simulink model "electrical_model"  (R2016a)
settings: Solver=VariableStepAuto  StartTime=0.0  StopTime=5  FixedStep=Ts  RelTol=1e-3
values from neighbouring files (symbols this model uses):
  Ts = 1    [MPC.m]
undefined symbols (not defined in the file or in its folder): Continuous, DiscIntNeverNeededParam, F, Li, ri, spsPMSynchronousMachineModel, w_g
libraries: powerlib x11, dspsrcs4 x6, powerlib_meascontrol x2, mpclib x1
settings Model: Creator=syf  LastModifiedBy=syf
settings SolverCC: AutoInsertRateTranBlk=on

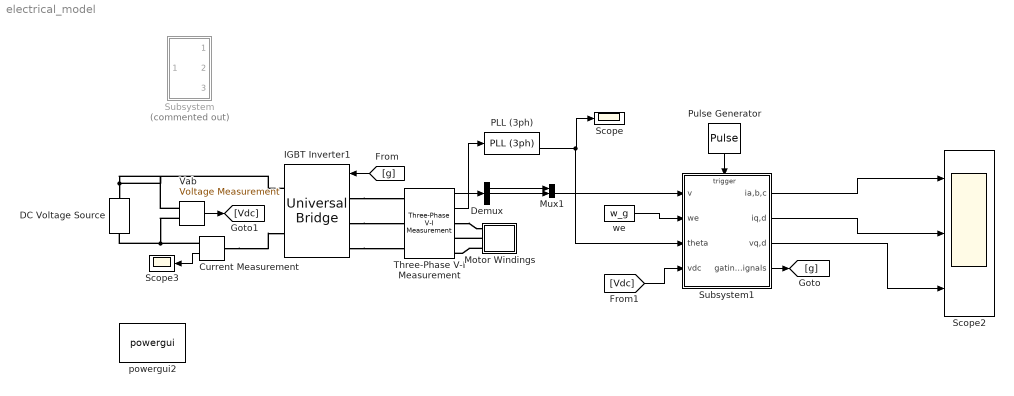
== system electrical_model ==
  Current Measurement : powerlib/Measurements/Current Measurement  PhasorSimulation=off  OutputType=Complex  PSBequivalent=0
  DC Voltage Source : powerlib/Electrical Sources/DC Voltage Source  Amplitude=540  Measurements=None
  Demux : Demux  Outputs=3
  IGBT Inverter1 : powerlib/Power Electronics/Universal Bridge  Arms=3  SnubberResistance=1e6  SnubberCapacitance=1e-9  Device=IGBT / Diodes  Ron=1e-3  Lon=0  ForwardVoltages="[  0.8  0.8  ]"  ForwardVoltage=.8  GTOparameters=[ 1e-6 , 1e-6 ]  IGBTparameters=[ 1e-6 , 2e-6 ]  Measurements=All voltages and currents  Measurements_2=None  converterType=Rectifier
  Motor Windings : Subsystem
  Mux1 : Mux  Inputs=2
  PLL (3ph) : powerlib_meascontrol/PLL/PLL (3ph)  Fmin=45  Par_Init=[0, 60]  ParK=[180, 3200, 1]  TcD=1e-4  MaxRateChangeFreq=12  FilterCutOffFreq=25  Ts=0  AGC=on
  Pulse Generator : DiscretePulseGenerator  PulseType=Time based  Period=Ts  PulseWidth=20
  Scope : Scope
  Scope2 : Scope  NumInputPorts=3
  Scope3 : Scope
  Subsystem : Subsystem  Commented=on
  Subsystem1 : Subsystem
  Three-Phase V-I Measurement : powerlib/Measurements/Three-Phase V-I Measurement  VoltageMeasurement=phase-to-phase  SetLabelV=off  LabelV=Vabc  Vpu=off  VpuLL=off  CurrentMeasurement=yes  SetLabelI=off  LabelI=Iabc  Ipu=off  Pbase=100e6  Vbase=500e3  OutputType=Complex  PhasorSimulation=off  PSBequivalent=0
  Vab : powerlib/Measurements/Voltage Measurement  Tag=PoWeRsYsTeMmEaSuReMeNt  PhasorSimulation=off  OutputType=Magnitude  PSBequivalent=0
  powergui2 : powerlib/powergui  Priority=1  SimulationMode=Continuous  SolverType=Backward Euler  SampleTime=Ts  frequency=60  SPID=off  DisableSnubberDevices=off  DisableRonSwitches=off  DisableVfSwitches=off  SwTol=0  DisplayEquations=off  Interpol=off  ExternalGateDelay=off  methode=off  Ts=10  FunctionMessages=off  echomessages=off  HookPort=off  EnableUseOfTLC=off  x0status=blocks  frequencyindice=0  Pbase=100e6  ErrMax=1e-4  Iterations=50  UnitsV=kV  UnitsW=MW  buscounter=0  RestoreLinks=warning  ResistiveCurrentMeasurement=off  Frange=[0:2:500]  Ylog=off  Xlog=on  ShowGrid=off  save=off  variable=ZData  structure=0  ZoomFFT=off  StartTime=0.0  cycles=1  DisplayStyle=1  fundamental=60  FreqAxis=off  MaxFrequency=1000  frequencyindicesteady=1  RmsSteady=1  display=off
  we : Constant  Value=w_g
  wires:
  Three-Phase V-I Measurement/1 -> Demux/1
  Demux/1 -> Mux1/1
  Demux/2 -> Mux1/2
  Vab/1 -> [Vdc]
  Current Measurement/1 -> Scope3/1
  Three-Phase V-I Measurement/2 -> PLL (3ph)/1
  PLL (3ph)/2 -> Subsystem1/3(theta), Scope/1
  [g] -> IGBT Inverter1/1
  Pulse Generator/1 -> Subsystem1/Trigger
  we/1 -> Subsystem1/2(we)
  [Vdc] -> Subsystem1/4(vdc)
  Subsystem1/4(gating signals) -> [g]
  Mux1/1 -> Subsystem1/1(v)
  Subsystem1/1(ia,b,c) -> Scope2/1
  Subsystem1/2(iq,d) -> Scope2/2
  Subsystem1/3(vq,d) -> Scope2/3
  connections:
  Current Measurement/RConn1 -- Vab/LConn2 -- DC Voltage Source/LConn1
  DC Voltage Source/RConn1 -- IGBT Inverter1/RConn1 -- Vab/LConn1
  Current Measurement/LConn1 -- IGBT Inverter1/RConn2
  IGBT Inverter1/LConn1 -- Three-Phase V-I Measurement/LConn1
  IGBT Inverter1/LConn2 -- Three-Phase V-I Measurement/LConn2
  IGBT Inverter1/LConn3 -- Three-Phase V-I Measurement/LConn3
  Three-Phase V-I Measurement/RConn1 -- Motor Windings/LConn1
  Motor Windings/LConn2 -- Three-Phase V-I Measurement/RConn2
  Motor Windings/LConn3 -- Three-Phase V-I Measurement/RConn3

== system electrical_model/Motor Windings ==
  phasea : powerlib/Elements/Series RLC Branch  LConnTagsString=__new0  RConnTagsString=__new0  BranchType=RL  Resistance=8e-3  Inductance=2.07e-3  SetiL0=off  InitialCurrent=0  Capacitance=0  Setx0=off  InitialVoltage=0  Measurements=None
  phaseb : powerlib/Elements/Series RLC Branch  LConnTagsString=__new0  RConnTagsString=__new0  BranchType=RL  Resistance=8e-3  Inductance=2.07e-3  SetiL0=off  InitialCurrent=0  Capacitance=0  Setx0=off  InitialVoltage=0  Measurements=None
  phasec : powerlib/Elements/Series RLC Branch  LConnTagsString=__new0  RConnTagsString=__new0  BranchType=RL  Resistance=8e-3  Inductance=2.07e-3  SetiL0=off  InitialCurrent=0  Capacitance=0  Setx0=off  InitialVoltage=0  Measurements=None
  A : PMIOPort  Port=1  Side=Left
  B : PMIOPort  Port=2  Side=Left
  C : PMIOPort  Port=3  Side=Left
  connections:
  phasea/RConn1 -- phasec/RConn1 -- phaseb/RConn1
  phaseb/LConn1 -- B/RConn1
  A/RConn1 -- phasea/LConn1
  phasec/LConn1 -- C/RConn1

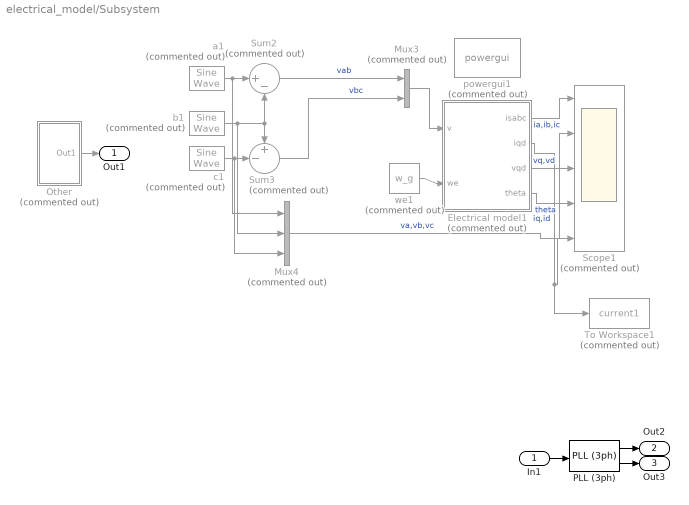
== system electrical_model/Subsystem ==
  In1 : Inport
  Electrical model1 : Subsystem  Commented=on  AncestorBlock=spsPMSynchronousMachineModel/Continuous
  Mux3 : Mux  Commented=on  Inputs=2
  Mux4 : Mux  Commented=on  Inputs=3
  Other : Subsystem  Commented=on
  PLL (3ph) : powerlib_meascontrol/PLL/PLL (3ph)  Fmin=45  Par_Init=[0, 60]  ParK=[180, 3200, 1]  TcD=1e-4  MaxRateChangeFreq=12  FilterCutOffFreq=25  Ts=0  AGC=on
  Scope1 : Scope  Commented=on  NumInputPorts=5
  Sum2 : Sum  Commented=on  Inputs=|+-
  Sum3 : Sum  Commented=on  Inputs=+-|
  To Workspace1 : ToWorkspace  Commented=on  VariableName=current1  SampleTime=-1
  a1 : dspsrcs4/Sine Wave  Commented=on  Amplitude=200  Frequency=w_g/(2*pi)  Phase=0  SampleMode=Discrete  OutComplex=Real  CompMethod=Trigonometric fcn  TableSize=Speed  SampleTime=Ts  SamplesPerFrame=1  ResetState=Restart at time zero  OutputFrames=off  dataType=double  wordLen=16  udDataType=sfix(16)  fracBitsMode=Best precision  numFracBits=15  OutDataTypeStr=double  LastOutDataTypeStr=double
  b1 : dspsrcs4/Sine Wave  Commented=on  Amplitude=200  Frequency=w_g/(2*pi)  Phase=2*pi/3  SampleMode=Discrete  OutComplex=Real  CompMethod=Trigonometric fcn  TableSize=Speed  SampleTime=Ts  SamplesPerFrame=1  ResetState=Restart at time zero  OutputFrames=off  dataType=double  wordLen=16  udDataType=sfix(16)  fracBitsMode=Best precision  numFracBits=15  OutDataTypeStr=double  LastOutDataTypeStr=double
  c1 : dspsrcs4/Sine Wave  Commented=on  Amplitude=200  Frequency=w_g/(2*pi)  Phase=-2*pi/3  SampleMode=Discrete  OutComplex=Real  CompMethod=Trigonometric fcn  TableSize=Speed  SampleTime=Ts  SamplesPerFrame=1  ResetState=Restart at time zero  OutputFrames=off  dataType=double  wordLen=16  udDataType=sfix(16)  fracBitsMode=Best precision  numFracBits=15  OutDataTypeStr=double  LastOutDataTypeStr=double
  powergui1 : powerlib/powergui  Priority=1  Commented=on  SimulationMode=Discrete  SolverType=Backward Euler  SampleTime=Ts  frequency=60  SPID=off  DisableSnubberDevices=off  DisableRonSwitches=off  DisableVfSwitches=off  SwTol=0  DisplayEquations=off  Interpol=off  ExternalGateDelay=off  methode=off  Ts=10  FunctionMessages=off  echomessages=off  HookPort=off  EnableUseOfTLC=off  x0status=blocks  frequencyindice=60  Pbase=100e6  ErrMax=1e-4  Iterations=50  UnitsV=kV  UnitsW=MW  buscounter=0  RestoreLinks=warning  ResistiveCurrentMeasurement=off  Frange=[0:2:500]  Ylog=off  Xlog=on  ShowGrid=off  save=off  variable=ZData  structure=0  ZoomFFT=off  StartTime=0.0  cycles=1  DisplayStyle=1  fundamental=60  FreqAxis=off  MaxFrequency=1000  frequencyindicesteady=1  RmsSteady=1  display=off
  we1 : Constant  Commented=on  Value=w_g
  Out1 : Outport
  Out2 : Outport  Port=2
  Out3 : Outport  Port=3
  wires:
  PLL (3ph)/2 -> Out3/1
  PLL (3ph)/1 -> Out2/1
  Other/1(Out1) -> Out1/1
  In1/1 -> PLL (3ph)/1
  we1/1 -> Electrical model1/2(we)
  Mux3/1 -> Electrical model1/1(v)
  Sum2/1 -> Mux3/1  "vab"
  Sum3/1 -> Mux3/2  "vbc"
  Electrical model1/1(isabc) -> Scope1/1  "ia,ib,ic"
  a1/1 -> Sum2/1, Mux4/1
  Electrical model1/2(iqd) -> To Workspace1/1, Scope1/5  "iq,id"
  c1/1 -> Sum3/2, Mux4/3
  Mux4/1 -> Scope1/2  "va,vb,vc"
  b1/1 -> Sum2/2, Sum3/1, Mux4/2
  Electrical model1/4(theta) -> Scope1/4  "theta"
  Electrical model1/3(vqd) -> Scope1/3  "vq,vd"

== system electrical_model/Subsystem1 ==
  v : Inport
  we : Inport  Port=2
  theta : Inport  Port=3
  vdc : Inport  Port=4
  Trigger : TriggerPort  VariantControl=Variant  PortDimensions=1
  Electrical model2 : Subsystem  AncestorBlock=spsPMSynchronousMachineModel/Continuous
  ia,b,c : Outport
  iq,d : Outport  Port=2
  vq,d : Outport  Port=3
  gating signals : Outport  Port=4
  wires:
  v/1 -> Electrical model2/1(v)
  we/1 -> Electrical model2/2(we)
  theta/1 -> Electrical model2/3(theta)
  Electrical model2/1(isabc) -> ia,b,c/1  "ia,ib,ic"
  Electrical model2/3(vqd) -> vq,d/1  "vq,vd"
  Electrical model2/4(Pulses) -> gating signals/1
  vdc/1 -> Electrical model2/4(Vdc)
  Electrical model2/2(iqd) -> iq,d/1  "iq,id"

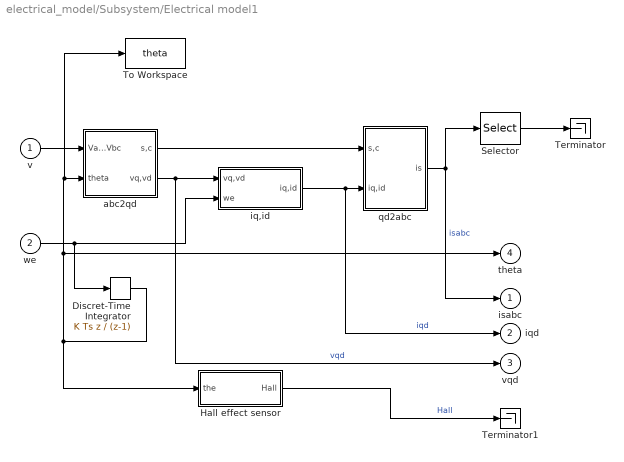
== system electrical_model/Subsystem/Electrical model1 ==
  v : Inport
  we : Inport  Port=2
  Discret-Time Integrator : DiscreteIntegrator  IntegratorMethod=Integration: Backward Euler  gainval=1  InitialConditionSetting=State (most efficient)  SampleTime=Ts  ICPrevOutput=DiscIntNeverNeededParam  ICPrevScaledInput=DiscIntNeverNeededParam
  Hall effect sensor : Subsystem
  Selector : Selector  InputPortWidth=3  IndexOptions=Index vector (dialog)  Indices=1:2  OutputSizes=1
  Terminator : Terminator
  Terminator1 : Terminator
  To Workspace : ToWorkspace  VariableName=theta  SampleTime=-1
      settings: Save2DSignal=2-D array (concatenate along first dimension)
  abc2qd : Subsystem
  iq,id : Subsystem
  qd2abc : Subsystem
  isabc : Outport  InitialOutput=0
  iqd : Outport  Port=2  InitialOutput=0
  vqd : Outport  Port=3  InitialOutput=0
  theta : Outport  Port=4  InitialOutput=0
  wires:
  we/1 -> Discret-Time Integrator/1, iq,id/2(we)
  Discret-Time Integrator/1 -> Hall effect sensor/1(the), theta/1, abc2qd/2(theta), To Workspace/1
  abc2qd/2(vq,vd) -> iq,id/1(vq,vd), vqd/1  "vqd"
  abc2qd/1(s,c) -> qd2abc/1(s,c)
  v/1 -> abc2qd/1(Vab,Vbc)
  iq,id/1(iq,id) -> qd2abc/2(iq,id), iqd/1  "iqd"
  qd2abc/1(is) -> Selector/1, isabc/1  "isabc"
  Selector/1 -> Terminator/1
  Hall effect sensor/1(Hall) -> Terminator1/1  "Hall"

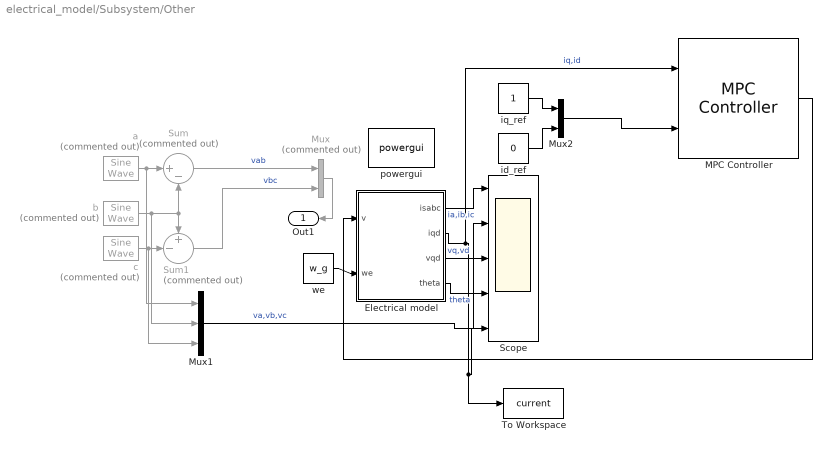
== system electrical_model/Subsystem/Other ==
  Electrical model : Subsystem  AncestorBlock=spsPMSynchronousMachineModel/Continuous
  MPC Controller : mpclib/MPC Controller  SCDEnableBlockLinearizationSpecification=on  is_multiple=0  enable_value=0  return_u0=off  ref_from_ws=off  ref_signal_name=[]  ref_preview=off  md_from_ws=off  md_signal_name=[]  md_preview=off  from_project=off  project_file=MPCtask.mat  md_inport=off  mv_inport=off  cost_outport=off  return_sequence=off  return_qpstatus=off  return_state=off  state_inport=off  lims_inport=off  ywt_inport=off  is_designfromscratch=0  uwt_inport=off  duwt_inport=off  rhoeps_inport=off  uref_inport=off  n_ts=1  n_mv=2  n_md=1  n_ud=0  n_mo=2  n_uo=0  BlockDataType=double  SampleTimeInherited=off  switch_inport=off
  Mux : Mux  Commented=on  Inputs=2
  Mux1 : Mux  Inputs=3
  Mux2 : Mux  Inputs=2
  Scope : Scope  NumInputPorts=5
  Sum : Sum  Commented=on  Inputs=|+-
  Sum1 : Sum  Commented=on  Inputs=+-|
  To Workspace : ToWorkspace  VariableName=current  SampleTime=-1
  a : dspsrcs4/Sine Wave  Commented=on  Amplitude=200  Frequency=w_g/(2*pi)  Phase=0  SampleMode=Discrete  OutComplex=Real  CompMethod=Trigonometric fcn  TableSize=Speed  SampleTime=Ts  SamplesPerFrame=1  ResetState=Restart at time zero  OutputFrames=off  dataType=double  wordLen=16  udDataType=sfix(16)  fracBitsMode=Best precision  numFracBits=15  OutDataTypeStr=double  LastOutDataTypeStr=double
  b : dspsrcs4/Sine Wave  Commented=on  Amplitude=200  Frequency=w_g/(2*pi)  Phase=2*pi/3  SampleMode=Discrete  OutComplex=Real  CompMethod=Trigonometric fcn  TableSize=Speed  SampleTime=Ts  SamplesPerFrame=1  ResetState=Restart at time zero  OutputFrames=off  dataType=double  wordLen=16  udDataType=sfix(16)  fracBitsMode=Best precision  numFracBits=15  OutDataTypeStr=double  LastOutDataTypeStr=double
  c : dspsrcs4/Sine Wave  Commented=on  Amplitude=200  Frequency=w_g/(2*pi)  Phase=-2*pi/3  SampleMode=Discrete  OutComplex=Real  CompMethod=Trigonometric fcn  TableSize=Speed  SampleTime=Ts  SamplesPerFrame=1  ResetState=Restart at time zero  OutputFrames=off  dataType=double  wordLen=16  udDataType=sfix(16)  fracBitsMode=Best precision  numFracBits=15  OutDataTypeStr=double  LastOutDataTypeStr=double
  id_ref : Constant  Value=0
  iq_ref : Constant
  powergui : powerlib/powergui  Priority=1  SimulationMode=Discrete  SolverType=Backward Euler  SampleTime=Ts  frequency=60  SPID=off  DisableSnubberDevices=off  DisableRonSwitches=off  DisableVfSwitches=off  SwTol=0  DisplayEquations=off  Interpol=off  ExternalGateDelay=off  methode=off  Ts=10  FunctionMessages=off  echomessages=off  HookPort=off  EnableUseOfTLC=off  x0status=blocks  frequencyindice=60  Pbase=100e6  ErrMax=1e-4  Iterations=50  UnitsV=kV  UnitsW=MW  buscounter=0  RestoreLinks=warning  ResistiveCurrentMeasurement=off  Frange=[0:2:500]  Ylog=off  Xlog=on  ShowGrid=off  save=off  variable=ZData  structure=0  ZoomFFT=off  StartTime=0.0  cycles=1  DisplayStyle=1  fundamental=60  FreqAxis=off  MaxFrequency=1000  frequencyindicesteady=1  RmsSteady=1  display=off
  we : Constant  Value=w_g
  Out1 : Outport
  wires:
  Electrical model/4(theta) -> Scope/4  "theta"
  Mux2/1 -> MPC Controller/2
  iq_ref/1 -> Mux2/1
  we/1 -> Electrical model/2(we)
  Sum/1 -> Mux/1  "vab"
  Electrical model/1(isabc) -> Scope/1  "ia,ib,ic"
  Electrical model/3(vqd) -> Scope/3  "vq,vd"
  Mux/1 -> Out1/1
  a/1 -> Mux1/1, Sum/1
  Electrical model/2(iqd) -> MPC Controller/1, Scope/5, To Workspace/1  "iq,id"
  b/1 -> Mux1/2, Sum1/1, Sum/2
  Sum1/1 -> Mux/2  "vbc"
  c/1 -> Mux1/3, Sum1/2
  Mux1/1 -> Scope/2  "va,vb,vc"
  MPC Controller/1 -> Electrical model/1(v)
  id_ref/1 -> Mux2/2

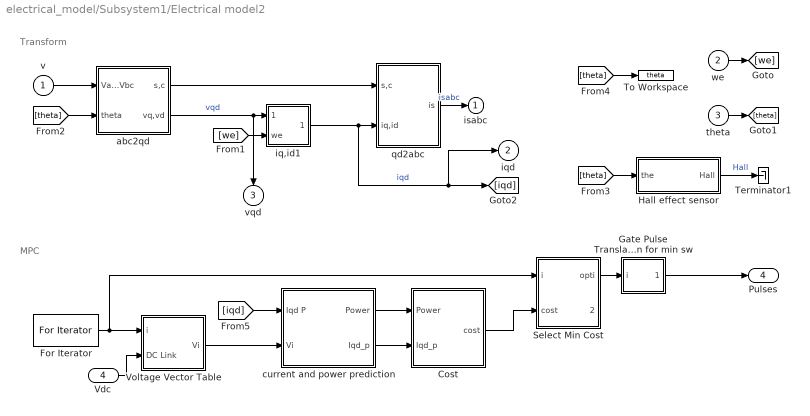
== system electrical_model/Subsystem1/Electrical model2 ==
  note: Transform
  note: MPC
  v : Inport
  we : Inport  Port=2
  theta : Inport  Port=3
  Vdc : Inport  Port=4
  "Cost " : Subsystem
  For Iterator : ForIterator  IterationLimit=7  IterationVariableDataType=double
  Gate Pulse Translation for min sw : Subsystem
  Hall effect sensor : Subsystem
  Select Min Cost : Subsystem
  Terminator1 : Terminator
  To Workspace : ToWorkspace  VariableName=theta  SampleTime=-1
      settings: Save2DSignal=2-D array (concatenate along first dimension)
  Voltage Vector Table : Subsystem
  abc2qd : Subsystem
  current and power prediction : Subsystem
  iq,id1 : Subsystem
  qd2abc : Subsystem
  isabc : Outport  InitialOutput=0
  iqd : Outport  Port=2  InitialOutput=0
  vqd : Outport  Port=3  InitialOutput=0
  Pulses : Outport  Port=4
  wires:
  Hall effect sensor/1(Hall) -> Terminator1/1  "Hall"
  qd2abc/1(is) -> isabc/1  "isabc"
  iq,id1/1(iq,id) -> iqd/1, [iqd], qd2abc/2(iq,id)  "iqd"
  v/1 -> abc2qd/1(Vab,Vbc)
  abc2qd/1(s,c) -> qd2abc/1(s,c)
  abc2qd/2(vq,vd) -> iq,id1/1(vq,vd), vqd/1  "vqd"
  Voltage Vector Table/1(Vi) -> current and power prediction/2(Vi)
  Vdc/1 -> Voltage Vector Table/2(DC Link)
  For Iterator/1 -> Select Min Cost/1(i), Voltage Vector Table/1(i)
  Gate Pulse Translation for min sw/1(pulses) -> Pulses/1
  Select Min Cost/1(opti) -> Gate Pulse Translation for min sw/1(i)
  we/1 -> [we]
  [we] -> iq,id1/2(we)
  theta/1 -> [theta]
  [theta] -> abc2qd/2(theta)
  [theta] -> Hall effect sensor/1(the)
  [theta] -> To Workspace/1
  [iqd] -> current and power prediction/1(Iqd P)
  current and power prediction/1(Power) -> "Cost "/1(Power)
  current and power prediction/2(Iqd_p) -> "Cost "/2("Iqd_p ")
  "Cost "/1(cost) -> Select Min Cost/2(cost)

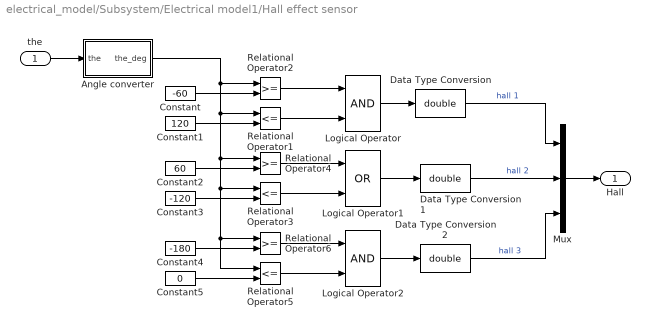
== system electrical_model/Subsystem/Electrical model1/Hall effect sensor ==
  the : Inport
  Angle converter : Subsystem
  Constant : Constant  Value=-60
  Constant1 : Constant  Value=120
  Constant2 : Constant  Value=60
  Constant3 : Constant  Value=-120
  Constant4 : Constant  Value=-180
  Constant5 : Constant  Value=0
  Data Type Conversion : DataTypeConversion  OutDataTypeStr=double  SaturateOnIntegerOverflow=on  RndMeth=Zero
  Data Type Conversion1 : DataTypeConversion  OutDataTypeStr=double  SaturateOnIntegerOverflow=on  RndMeth=Zero
  Data Type Conversion2 : DataTypeConversion  OutDataTypeStr=double  SaturateOnIntegerOverflow=on  RndMeth=Zero
  Logical Operator : Logic  AllPortsSameDT=off  OutDataTypeStr=boolean
  Logical Operator1 : Logic  Operator=OR  AllPortsSameDT=off  OutDataTypeStr=boolean
  Logical Operator2 : Logic  AllPortsSameDT=off  OutDataTypeStr=boolean
  Mux : Mux  Inputs=3
  Relational Operator1 : RelationalOperator  Operator=<=  InputSameDT=on
  Relational Operator2 : RelationalOperator  InputSameDT=on
  Relational Operator3 : RelationalOperator  Operator=<=  InputSameDT=on
  Relational Operator4 : RelationalOperator  InputSameDT=on
  Relational Operator5 : RelationalOperator  Operator=<=  InputSameDT=on
  Relational Operator6 : RelationalOperator  InputSameDT=on
  Hall : Outport
  wires:
  the/1 -> Angle converter/1(the)
  Constant3/1 -> Relational Operator3/2
  Constant2/1 -> Relational Operator4/2
  Relational Operator4/1 -> Logical Operator1/1
  Constant1/1 -> Relational Operator1/2
  Constant/1 -> Relational Operator2/2
  Angle converter/1(the_deg) -> Relational Operator4/1, Relational Operator3/1, Relational Operator5/1, Relational Operator6/1, Relational Operator1/1, Relational Operator2/1
  Relational Operator1/1 -> Logical Operator/2
  Relational Operator2/1 -> Logical Operator/1
  Logical Operator/1 -> Data Type Conversion/1
  Logical Operator1/1 -> Data Type Conversion1/1
  Relational Operator3/1 -> Logical Operator1/2
  Constant5/1 -> Relational Operator5/2
  Constant4/1 -> Relational Operator6/2
  Relational Operator6/1 -> Logical Operator2/1
  Logical Operator2/1 -> Data Type Conversion2/1
  Relational Operator5/1 -> Logical Operator2/2
  Data Type Conversion/1 -> Mux/1  "hall 1"
  Data Type Conversion1/1 -> Mux/2  "hall 2"
  Data Type Conversion2/1 -> Mux/3  "hall 3"
  Mux/1 -> Hall/1

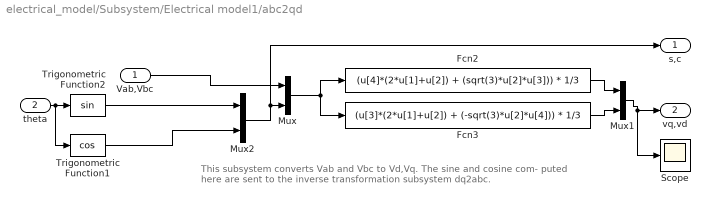
== system electrical_model/Subsystem/Electrical model1/abc2qd ==
  note: This subsystem converts Vab and Vbc to Vd,Vq. The sine and cosine com-
      | puted here are sent to the inverse transformation subsystem dq2abc.
  Vab,Vbc : Inport
  theta : Inport  Port=2
  Fcn2 : Fcn  Expr=(u[4]*(2*u[1]+u[2]) + (sqrt(3)*u[2]*u[3])) * 1/3
  Fcn3 : Fcn  Expr=(u[3]*(2*u[1]+u[2]) + (-sqrt(3)*u[2]*u[4])) * 1/3
  Mux : Mux  Inputs=2
  Mux1 : Mux  Inputs=2
  Mux2 : Mux  Inputs=2
  Scope : Scope
  Trigonometric Function1 : Trigonometry  Operator=cos  SampleTime=Ts
  Trigonometric Function2 : Trigonometry  SampleTime=Ts
  s,c : Outport  InitialOutput=0
  vq,vd : Outport  Port=2  InitialOutput=0
  wires:
  theta/1 -> Trigonometric Function2/1, Trigonometric Function1/1
  Trigonometric Function1/1 -> Mux2/2
  Trigonometric Function2/1 -> Mux2/1
  Fcn3/1 -> Mux1/2
  Mux/1 -> Fcn2/1, Fcn3/1
  Mux2/1 -> s,c/1, Mux/2
  Fcn2/1 -> Mux1/1
  Mux1/1 -> vq,vd/1, Scope/1
  Vab,Vbc/1 -> Mux/1

== system electrical_model/Subsystem/Electrical model1/iq,id ==
  vq,vd : Inport
  we : Inport  Port=2
  Demux : Demux  Outputs=2
  Mux : Mux  Inputs=2
  Scope : Scope  NumInputPorts=2
  id : Subsystem
  iq : Subsystem
  iq,id : Outport  InitialOutput=0
  wires:
  id/1(id) -> Mux/2, Scope/2, iq/3(id)
  we/1 -> iq/2(we), id/2(we)
  iq/1(iq) -> Mux/1, id/3(iq), Scope/1  "i"
  Demux/2 -> id/1(vd)
  Demux/1 -> iq/1(vq)  "v"
  vq,vd/1 -> Demux/1
  Mux/1 -> iq,id/1

== system electrical_model/Subsystem/Electrical model1/qd2abc ==
  s,c : Inport
  iq,id : Inport  Port=2
  Fcn : Fcn  Expr=u[3]*u[2] + u[4]*u[1]
  Fcn1 : Fcn  Expr=(u[2]*(-u[3]-sqrt(3)*u[4]) + u[1]*(sqrt(3)*u[3]-u[4]))*0.5
  Mux1 : Mux  Inputs=2
  Mux3 : Mux  Inputs=3
  Sum : Sum  Inputs=--  SaturateOnIntegerOverflow=on  InputSameDT=on  OutDataTypeStr=Inherit: Same as first input
  is : Outport  InitialOutput=0
  wires:
  Mux1/1 -> Fcn/1, Fcn1/1
  s,c/1 -> Mux1/1
  iq,id/1 -> Mux1/2
  Sum/1 -> Mux3/3
  Fcn/1 -> Sum/2, Mux3/1
  Fcn1/1 -> Sum/1, Mux3/2
  Mux3/1 -> is/1

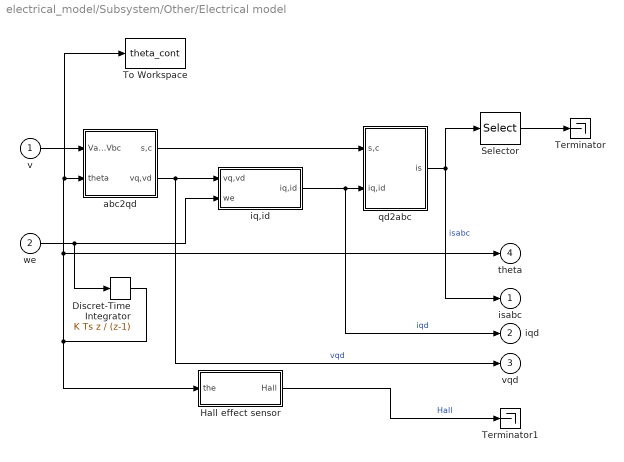
== system electrical_model/Subsystem/Other/Electrical model ==
  v : Inport
  we : Inport  Port=2
  Discret-Time Integrator : DiscreteIntegrator  IntegratorMethod=Integration: Backward Euler  gainval=1  InitialConditionSetting=State (most efficient)  SampleTime=Ts  ICPrevOutput=DiscIntNeverNeededParam  ICPrevScaledInput=DiscIntNeverNeededParam
  Hall effect sensor : Subsystem
  Selector : Selector  InputPortWidth=3  IndexOptions=Index vector (dialog)  Indices=1:2  OutputSizes=1
  Terminator : Terminator
  Terminator1 : Terminator
  To Workspace : ToWorkspace  VariableName=theta_cont  SampleTime=-1
      settings: Save2DSignal=2-D array (concatenate along first dimension)
  abc2qd : Subsystem
  iq,id : Subsystem
  qd2abc : Subsystem
  isabc : Outport  InitialOutput=0
  iqd : Outport  Port=2  InitialOutput=0
  vqd : Outport  Port=3  InitialOutput=0
  theta : Outport  Port=4  InitialOutput=0
  wires:
  Hall effect sensor/1(Hall) -> Terminator1/1  "Hall"
  Selector/1 -> Terminator/1
  qd2abc/1(is) -> isabc/1, Selector/1  "isabc"
  iq,id/1(iq,id) -> iqd/1, qd2abc/2(iq,id)  "iqd"
  v/1 -> abc2qd/1(Vab,Vbc)
  abc2qd/1(s,c) -> qd2abc/1(s,c)
  abc2qd/2(vq,vd) -> vqd/1, iq,id/1(vq,vd)  "vqd"
  Discret-Time Integrator/1 -> To Workspace/1, abc2qd/2(theta), theta/1, Hall effect sensor/1(the)
  we/1 -> iq,id/2(we), Discret-Time Integrator/1

== system electrical_model/Subsystem1/Electrical model2/Cost  ==
  Power : Inport
  "Iqd_p " : Inport  Port=2
  cost : Outport
  wires:
  Power/1 -> cost/1

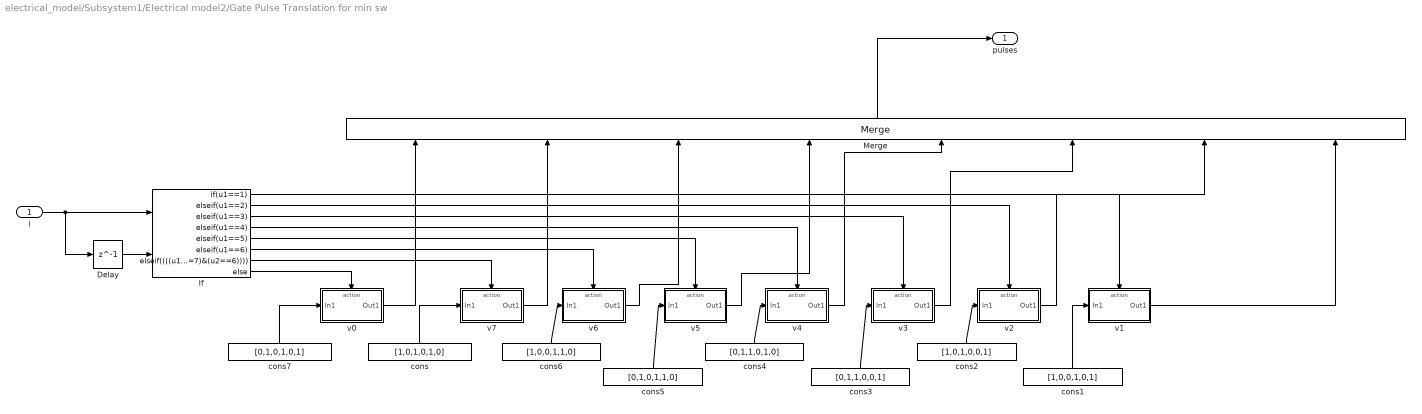
== system electrical_model/Subsystem1/Electrical model2/Gate Pulse Translation for min sw ==
  i : Inport
  Delay : Delay  DelayLength=1  InitialCondition=0
  If : If  NumInputs=2  IfExpression=u1==1  ElseIfExpressions=u1==2, u1==3, u1==4, u1==5, u1==6,(((u1==7)&(u2==2)) | ((u1==7)&(u2==4)) | ((u1==7)&(u2==6)))
  Merge : Merge  Inputs=8
  cons : Constant  Value=[1,0,1,0,1,0]
  cons1 : Constant  Value=[1,0,0,1,0,1]
  cons2 : Constant  Value=[1,0,1,0,0,1]
  cons3 : Constant  Value=[0,1,1,0,0,1]
  cons4 : Constant  Value=[0,1,1,0,1,0]
  cons5 : Constant  Value=[0,1,0,1,1,0]
  cons6 : Constant  Value=[1,0,0,1,1,0]
  cons7 : Constant  Value=[0,1,0,1,0,1]
  v0 : Subsystem  TreatAsAtomicUnit=on
  v1 : Subsystem  TreatAsAtomicUnit=on
  v2 : Subsystem  TreatAsAtomicUnit=on
  v3 : Subsystem  TreatAsAtomicUnit=on
  v4 : Subsystem  TreatAsAtomicUnit=on
  v5 : Subsystem  TreatAsAtomicUnit=on
  v6 : Subsystem  TreatAsAtomicUnit=on
  v7 : Subsystem  TreatAsAtomicUnit=on
  pulses : Outport
  wires:
  i/1 -> Delay/1, If/1
  If/1 -> v1/Action
  Merge/1 -> pulses/1
  cons/1 -> v7/1(In1)
  If/3 -> v3/Action
  If/2 -> v2/Action
  If/4 -> v4/Action
  If/5 -> v5/Action
  If/7 -> v7/Action
  If/6 -> v6/Action
  cons1/1 -> v1/1(In1)
  cons2/1 -> v2/1(In1)
  cons3/1 -> v3/1(In1)
  cons4/1 -> v4/1(In1)
  cons5/1 -> v5/1(In1)
  cons6/1 -> v6/1(In1)
  Delay/1 -> If/2
  cons7/1 -> v0/1(In1)
  If/8 -> v0/Action
  v0/1(Out1) -> Merge/1
  v7/1(Out1) -> Merge/2
  v6/1(Out1) -> Merge/3
  v5/1(Out1) -> Merge/4
  v4/1(Out1) -> Merge/5
  v3/1(Out1) -> Merge/6
  v2/1(Out1) -> Merge/7
  v1/1(Out1) -> Merge/8

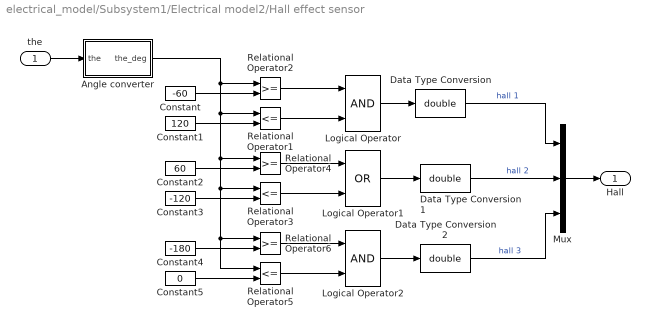
== system electrical_model/Subsystem1/Electrical model2/Hall effect sensor ==
  the : Inport
  Angle converter : Subsystem
  Constant : Constant  Value=-60
  Constant1 : Constant  Value=120
  Constant2 : Constant  Value=60
  Constant3 : Constant  Value=-120
  Constant4 : Constant  Value=-180
  Constant5 : Constant  Value=0
  Data Type Conversion : DataTypeConversion  OutDataTypeStr=double  SaturateOnIntegerOverflow=on  RndMeth=Zero
  Data Type Conversion1 : DataTypeConversion  OutDataTypeStr=double  SaturateOnIntegerOverflow=on  RndMeth=Zero
  Data Type Conversion2 : DataTypeConversion  OutDataTypeStr=double  SaturateOnIntegerOverflow=on  RndMeth=Zero
  Logical Operator : Logic  AllPortsSameDT=off  OutDataTypeStr=boolean
  Logical Operator1 : Logic  Operator=OR  AllPortsSameDT=off  OutDataTypeStr=boolean
  Logical Operator2 : Logic  AllPortsSameDT=off  OutDataTypeStr=boolean
  Mux : Mux  Inputs=3
  Relational Operator1 : RelationalOperator  Operator=<=  InputSameDT=on
  Relational Operator2 : RelationalOperator  InputSameDT=on
  Relational Operator3 : RelationalOperator  Operator=<=  InputSameDT=on
  Relational Operator4 : RelationalOperator  InputSameDT=on
  Relational Operator5 : RelationalOperator  Operator=<=  InputSameDT=on
  Relational Operator6 : RelationalOperator  InputSameDT=on
  Hall : Outport
  wires:
  Mux/1 -> Hall/1
  Data Type Conversion2/1 -> Mux/3  "hall 3"
  Data Type Conversion1/1 -> Mux/2  "hall 2"
  Data Type Conversion/1 -> Mux/1  "hall 1"
  Relational Operator5/1 -> Logical Operator2/2
  Logical Operator2/1 -> Data Type Conversion2/1
  Relational Operator6/1 -> Logical Operator2/1
  Constant4/1 -> Relational Operator6/2
  Constant5/1 -> Relational Operator5/2
  Relational Operator3/1 -> Logical Operator1/2
  Logical Operator1/1 -> Data Type Conversion1/1
  Logical Operator/1 -> Data Type Conversion/1
  Relational Operator2/1 -> Logical Operator/1
  Relational Operator1/1 -> Logical Operator/2
  Angle converter/1(the_deg) -> Relational Operator2/1, Relational Operator1/1, Relational Operator6/1, Relational Operator5/1, Relational Operator3/1, Relational Operator4/1
  Constant/1 -> Relational Operator2/2
  Constant1/1 -> Relational Operator1/2
  Relational Operator4/1 -> Logical Operator1/1
  Constant2/1 -> Relational Operator4/2
  Constant3/1 -> Relational Operator3/2
  the/1 -> Angle converter/1(the)

== system electrical_model/Subsystem1/Electrical model2/Select Min Cost ==
  i : Inport
  cost : Inport  Port=2
  Demux2 : Demux  Outputs=2
  If1 : If  NumInputs=3  IfExpression=u1==1  ElseIfExpressions=u2<=u3  ShowElse=off
  Merge1 : Merge
  Mux6 : Mux  Inputs=2
  Unit Delay : UnitDelay  SampleTime=-1
  v7 and v1 : Subsystem  TreatAsAtomicUnit=on
  v7 and v2 : Subsystem  TreatAsAtomicUnit=on
  opti : Outport
  mincost : Outport  Port=2
  wires:
  cost/1 -> Mux6/2, If1/2
  If1/1 -> v7 and v2/Action
  Unit Delay/1 -> If1/3
  i/1 -> Mux6/1, If1/1
  Mux6/1 -> v7 and v1/1(In1), v7 and v2/1(In1)
  Merge1/1 -> Demux2/1
  Demux2/2 -> mincost/1, Unit Delay/1
  If1/2 -> v7 and v1/Action
  v7 and v1/1(Out1) -> Merge1/1
  v7 and v2/1(Out1) -> Merge1/2
  Demux2/1 -> opti/1

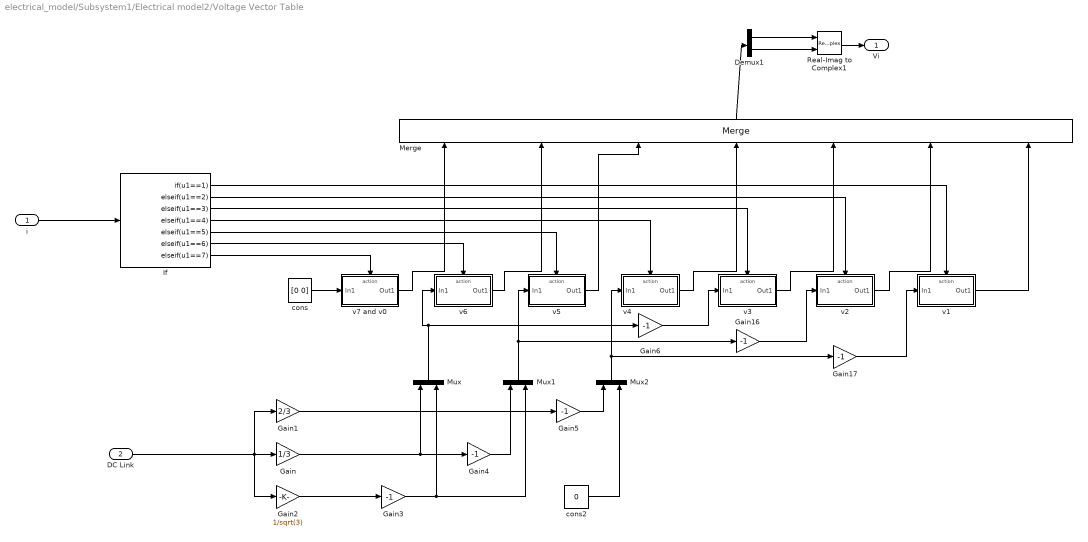
== system electrical_model/Subsystem1/Electrical model2/Voltage Vector Table ==
  i : Inport
  DC Link : Inport  Port=2
  Demux1 : Demux  Outputs=2
  Gain : Gain  Gain=1/3
  Gain1 : Gain  Gain=2/3
  Gain{3..6,16..17} (6 alike) : Gain  Gain=-1
  Gain2 : Gain  Gain=1/sqrt(3)
  If : If  IfExpression=u1==1  ElseIfExpressions=u1==2, u1==3, u1==4, u1==5, u1==6, u1==7  ShowElse=off
  Merge : Merge  Inputs=7
  Mux : Mux  Inputs=2
  Mux1 : Mux  Inputs=2
  Mux2 : Mux  Inputs=2
  Real-Imag to Complex1 : RealImagToComplex
  cons : Constant  Value=[0 0]
  cons2 : Constant  Value=0
  v1 : Subsystem  TreatAsAtomicUnit=on
  v2 : Subsystem  TreatAsAtomicUnit=on
  v3 : Subsystem  TreatAsAtomicUnit=on
  v4 : Subsystem  TreatAsAtomicUnit=on
  v5 : Subsystem  TreatAsAtomicUnit=on
  v6 : Subsystem  TreatAsAtomicUnit=on
  v7 and v0 : Subsystem  TreatAsAtomicUnit=on
  Vi : Outport
  wires:
  i/1 -> If/1
  Gain16/1 -> v2/1(In1)
  Gain6/1 -> v3/1(In1)
  Gain17/1 -> v1/1(In1)
  If/1 -> v1/Action
  Gain4/1 -> Mux1/1
  cons2/1 -> Mux2/2
  Merge/1 -> Demux1/1
  Gain1/1 -> Gain5/1
  cons/1 -> v7 and v0/1(In1)
  Gain2/1 -> Gain3/1
  Gain3/1 -> Mux1/2, Mux/2
  DC Link/1 -> Gain1/1, Gain/1, Gain2/1
  Mux2/1 -> Gain17/1, v4/1(In1)
  Mux1/1 -> Gain16/1, v5/1(In1)
  If/3 -> v3/Action
  Mux/1 -> Gain6/1, v6/1(In1)
  Demux1/2 -> Real-Imag to Complex1/2
  Gain5/1 -> Mux2/1
  If/2 -> v2/Action
  If/4 -> v4/Action
  If/5 -> v5/Action
  If/7 -> v7 and v0/Action
  Demux1/1 -> Real-Imag to Complex1/1
  If/6 -> v6/Action
  Gain/1 -> Gain4/1, Mux/1
  Real-Imag to Complex1/1 -> Vi/1
  v1/1(Out1) -> Merge/7
  v2/1(Out1) -> Merge/6
  v3/1(Out1) -> Merge/5
  v4/1(Out1) -> Merge/4
  v5/1(Out1) -> Merge/3
  v6/1(Out1) -> Merge/2
  v7 and v0/1(Out1) -> Merge/1

== system electrical_model/Subsystem1/Electrical model2/abc2qd ==
  note: This subsystem converts Vab and Vbc to Vd,Vq. The sine and cosine com-
      | puted here are sent to the inverse transformation subsystem dq2abc.
  Vab,Vbc : Inport
  theta : Inport  Port=2
  Fcn2 : Fcn  Expr=(u[4]*(2*u[1]+u[2]) + (sqrt(3)*u[2]*u[3])) * 1/3
  Fcn3 : Fcn  Expr=(u[3]*(2*u[1]+u[2]) + (-sqrt(3)*u[2]*u[4])) * 1/3
  Mux : Mux  Inputs=2
  Mux1 : Mux  Inputs=2
  Mux2 : Mux  Inputs=2
  Scope : Scope
  Trigonometric Function1 : Trigonometry  Operator=cos
  Trigonometric Function2 : Trigonometry
  s,c : Outport  InitialOutput=0
  vq,vd : Outport  Port=2  InitialOutput=0
  wires:
  Vab,Vbc/1 -> Mux/1
  Mux1/1 -> Scope/1, vq,vd/1
  Fcn2/1 -> Mux1/1
  Mux2/1 -> Mux/2, s,c/1
  Mux/1 -> Fcn3/1, Fcn2/1
  Fcn3/1 -> Mux1/2
  Trigonometric Function2/1 -> Mux2/1
  Trigonometric Function1/1 -> Mux2/2
  theta/1 -> Trigonometric Function1/1, Trigonometric Function2/1

== system electrical_model/Subsystem1/Electrical model2/current and power prediction ==
  Iqd P : Inport
  Vi : Inport  Port=2
  To Workspace : ToWorkspace  VariableName=IqId  SampleTime=-1
      settings: Save2DSignal=2-D array (concatenate along first dimension)
  cost function : MATLAB Function  TreatAsAtomicUnit=on
  Power : Outport
  Iqd_p : Outport  Port=2
  wires:
  Iqd P/1 -> cost function/1(u), To Workspace/1
  cost function/1(P) -> Power/1
  cost function/2(Iqd_next) -> Iqd_p/1

== system electrical_model/Subsystem1/Electrical model2/iq,id1 ==
  vq,vd : Inport
  we : Inport  Port=2
  Demux : Demux  Outputs=2
  Mux : Mux  Inputs=2
  id : Subsystem
  iq : Subsystem
  iq,id : Outport  InitialOutput=0
  wires:
  we/1 -> iq/2(we), id/2(we)
  id/1(id) -> Mux/2, iq/3(id)
  iq/1(iq) -> Mux/1, id/1(iq)
  Demux/2 -> id/3(vd)
  Demux/1 -> iq/1(vq)
  vq,vd/1 -> Demux/1
  Mux/1 -> iq,id/1

== system electrical_model/Subsystem1/Electrical model2/qd2abc ==
  s,c : Inport
  iq,id : Inport  Port=2
  Fcn : Fcn  Expr=u[3]*u[2] + u[4]*u[1]
  Fcn1 : Fcn  Expr=(u[2]*(-u[3]-sqrt(3)*u[4]) + u[1]*(sqrt(3)*u[3]-u[4]))*0.5
  Mux1 : Mux  Inputs=2
  Mux3 : Mux  Inputs=3
  Sum : Sum  Inputs=--  SaturateOnIntegerOverflow=on  InputSameDT=on  OutDataTypeStr=Inherit: Same as first input
  is : Outport  InitialOutput=0
  wires:
  Mux3/1 -> is/1
  Fcn1/1 -> Mux3/2, Sum/1
  Fcn/1 -> Mux3/1, Sum/2
  Sum/1 -> Mux3/3
  iq,id/1 -> Mux1/2
  s,c/1 -> Mux1/1
  Mux1/1 -> Fcn1/1, Fcn/1

== system electrical_model/Subsystem/Electrical model1/Hall effect sensor/Angle converter ==
  note: This subsystem convert 0,infinite angle to -180,180 angle
  the : Inport
  Trigonometric Function : Trigonometry
  Trigonometric Function1 : Trigonometry  Operator=cos
  Trigonometric Function2 : Trigonometry  Operator=atan2
  rad2deg : Gain  Gain=180/pi  SaturateOnIntegerOverflow=on  OutDataTypeStr=Inherit: Same as input  ParamDataTypeStr=Inherit: Same as input
  the_deg : Outport
  wires:
  rad2deg/1 -> the_deg/1
  Trigonometric Function2/1 -> rad2deg/1
  Trigonometric Function1/1 -> Trigonometric Function2/2
  Trigonometric Function/1 -> Trigonometric Function2/1
  the/1 -> Trigonometric Function1/1, Trigonometric Function/1

== system electrical_model/Subsystem/Electrical model1/iq,id/id ==
  vd : Inport
  we : Inport  Port=2
  iq : Inport  Port=3
  1-Ri/Li*Ts : Gain  Gain=1-ri/Li*Ts  SaturateOnIntegerOverflow=on  OutDataTypeStr=Inherit: Same as input  ParamDataTypeStr=Inherit: Same as input
  Product1 : Product  SaturateOnIntegerOverflow=on  InputSameDT=on  OutDataTypeStr=Inherit: Same as first input
  Sum1 : Sum  Inputs=-++  SaturateOnIntegerOverflow=on  InputSameDT=on  OutDataTypeStr=Inherit: Same as first input
  Ts : Gain  Gain=Ts  SaturateOnIntegerOverflow=on  OutDataTypeStr=Inherit: Same as input  ParamDataTypeStr=Inherit: Same as input
  Ts/Li : Gain  Gain=Ts/Li  SaturateOnIntegerOverflow=on  OutDataTypeStr=Inherit: Same as input  ParamDataTypeStr=Inherit: Same as input
  Unit Delay : UnitDelay  SampleTime=-1
  id : Outport  InitialOutput=0
  wires:
  Unit Delay/1 -> 1-Ri/Li*Ts/1, id/1
  we/1 -> Product1/2
  vd/1 -> Ts/Li/1
  iq/1 -> Product1/1
  Ts/Li/1 -> Sum1/3
  Product1/1 -> Ts/1
  Sum1/1 -> Unit Delay/1  "idot"
  Ts/1 -> Sum1/2
  1-Ri/Li*Ts/1 -> Sum1/1

== system electrical_model/Subsystem/Electrical model1/iq,id/iq ==
  vq : Inport
  we : Inport  Port=2
  id : Inport  Port=3
  1-Ri/Li*Ts : Gain  Gain=1-ri/Li*Ts  SaturateOnIntegerOverflow=on  OutDataTypeStr=Inherit: Same as input  ParamDataTypeStr=Inherit: Same as input
  Product1 : Product  SaturateOnIntegerOverflow=on  InputSameDT=on  OutDataTypeStr=Inherit: Same as first input
  Sum1 : Sum  Inputs=--+  SaturateOnIntegerOverflow=on  InputSameDT=on  OutDataTypeStr=Inherit: Same as first input
  Ts : Gain  Gain=Ts  SaturateOnIntegerOverflow=on  OutDataTypeStr=Inherit: Same as input  ParamDataTypeStr=Inherit: Same as input
  Ts/Li : Gain  Gain=Ts/Li  SaturateOnIntegerOverflow=on  OutDataTypeStr=Inherit: Same as input  ParamDataTypeStr=Inherit: Same as input
  Unit Delay : UnitDelay  SampleTime=-1
  iq : Outport  InitialOutput=0
  wires:
  Unit Delay/1 -> iq/1, 1-Ri/Li*Ts/1
  we/1 -> Product1/2
  vq/1 -> Ts/Li/1
  id/1 -> Product1/1
  Ts/Li/1 -> Sum1/3
  Product1/1 -> Ts/1
  Sum1/1 -> Unit Delay/1  "idot"
  Ts/1 -> Sum1/2
  1-Ri/Li*Ts/1 -> Sum1/1

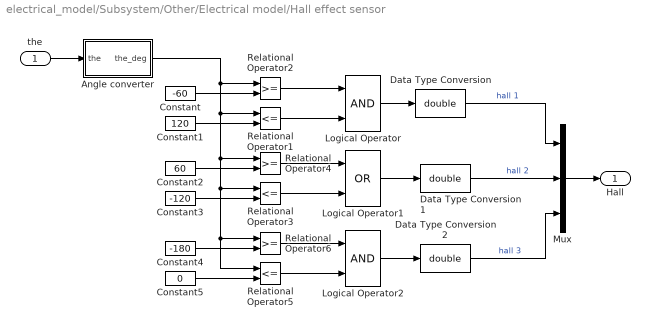
== system electrical_model/Subsystem/Other/Electrical model/Hall effect sensor ==
  the : Inport
  Angle converter : Subsystem
  Constant : Constant  Value=-60
  Constant1 : Constant  Value=120
  Constant2 : Constant  Value=60
  Constant3 : Constant  Value=-120
  Constant4 : Constant  Value=-180
  Constant5 : Constant  Value=0
  Data Type Conversion : DataTypeConversion  OutDataTypeStr=double  SaturateOnIntegerOverflow=on  RndMeth=Zero
  Data Type Conversion1 : DataTypeConversion  OutDataTypeStr=double  SaturateOnIntegerOverflow=on  RndMeth=Zero
  Data Type Conversion2 : DataTypeConversion  OutDataTypeStr=double  SaturateOnIntegerOverflow=on  RndMeth=Zero
  Logical Operator : Logic  AllPortsSameDT=off  OutDataTypeStr=boolean
  Logical Operator1 : Logic  Operator=OR  AllPortsSameDT=off  OutDataTypeStr=boolean
  Logical Operator2 : Logic  AllPortsSameDT=off  OutDataTypeStr=boolean
  Mux : Mux  Inputs=3
  Relational Operator1 : RelationalOperator  Operator=<=  InputSameDT=on
  Relational Operator2 : RelationalOperator  InputSameDT=on
  Relational Operator3 : RelationalOperator  Operator=<=  InputSameDT=on
  Relational Operator4 : RelationalOperator  InputSameDT=on
  Relational Operator5 : RelationalOperator  Operator=<=  InputSameDT=on
  Relational Operator6 : RelationalOperator  InputSameDT=on
  Hall : Outport
  wires:
  Mux/1 -> Hall/1
  Data Type Conversion2/1 -> Mux/3  "hall 3"
  Data Type Conversion1/1 -> Mux/2  "hall 2"
  Data Type Conversion/1 -> Mux/1  "hall 1"
  Relational Operator5/1 -> Logical Operator2/2
  Logical Operator2/1 -> Data Type Conversion2/1
  Relational Operator6/1 -> Logical Operator2/1
  Constant4/1 -> Relational Operator6/2
  Constant5/1 -> Relational Operator5/2
  Relational Operator3/1 -> Logical Operator1/2
  Logical Operator1/1 -> Data Type Conversion1/1
  Logical Operator/1 -> Data Type Conversion/1
  Relational Operator2/1 -> Logical Operator/1
  Relational Operator1/1 -> Logical Operator/2
  Angle converter/1(the_deg) -> Relational Operator2/1, Relational Operator1/1, Relational Operator6/1, Relational Operator5/1, Relational Operator3/1, Relational Operator4/1
  Constant/1 -> Relational Operator2/2
  Constant1/1 -> Relational Operator1/2
  Relational Operator4/1 -> Logical Operator1/1
  Constant2/1 -> Relational Operator4/2
  Constant3/1 -> Relational Operator3/2
  the/1 -> Angle converter/1(the)

== system electrical_model/Subsystem/Other/Electrical model/abc2qd ==
  note: This subsystem converts Vab and Vbc to Vd,Vq. The sine and cosine com-
      | puted here are sent to the inverse transformation subsystem dq2abc.
  Vab,Vbc : Inport
  theta : Inport  Port=2
  Fcn2 : Fcn  Expr=(u[4]*(2*u[1]+u[2]) + (sqrt(3)*u[2]*u[3])) * 1/3
  Fcn3 : Fcn  Expr=(u[3]*(2*u[1]+u[2]) + (-sqrt(3)*u[2]*u[4])) * 1/3
  Mux : Mux  Inputs=2
  Mux1 : Mux  Inputs=2
  Mux2 : Mux  Inputs=2
  Scope : Scope
  Trigonometric Function1 : Trigonometry  Operator=cos  SampleTime=Ts
  Trigonometric Function2 : Trigonometry  SampleTime=Ts
  s,c : Outport  InitialOutput=0
  vq,vd : Outport  Port=2  InitialOutput=0
  wires:
  Vab,Vbc/1 -> Mux/1
  Mux1/1 -> Scope/1, vq,vd/1
  Fcn2/1 -> Mux1/1
  Mux2/1 -> Mux/2, s,c/1
  Mux/1 -> Fcn3/1, Fcn2/1
  Fcn3/1 -> Mux1/2
  Trigonometric Function2/1 -> Mux2/1
  Trigonometric Function1/1 -> Mux2/2
  theta/1 -> Trigonometric Function1/1, Trigonometric Function2/1

== system electrical_model/Subsystem/Other/Electrical model/iq,id ==
  vq,vd : Inport
  we : Inport  Port=2
  Demux : Demux  Outputs=2
  Mux : Mux  Inputs=2
  Scope : Scope  NumInputPorts=2
  id : Subsystem
  iq : Subsystem
  iq,id : Outport  InitialOutput=0
  wires:
  Mux/1 -> iq,id/1
  vq,vd/1 -> Demux/1
  Demux/1 -> iq/1(vq)  "v"
  Demux/2 -> id/1(vd)
  iq/1(iq) -> Scope/1, id/3(iq), Mux/1  "i"
  we/1 -> id/2(we), iq/2(we)
  id/1(id) -> iq/3(id), Scope/2, Mux/2

== system electrical_model/Subsystem/Other/Electrical model/qd2abc ==
  s,c : Inport
  iq,id : Inport  Port=2
  Fcn : Fcn  Expr=u[3]*u[2] + u[4]*u[1]
  Fcn1 : Fcn  Expr=(u[2]*(-u[3]-sqrt(3)*u[4]) + u[1]*(sqrt(3)*u[3]-u[4]))*0.5
  Mux1 : Mux  Inputs=2
  Mux3 : Mux  Inputs=3
  Sum : Sum  Inputs=--  SaturateOnIntegerOverflow=on  InputSameDT=on  OutDataTypeStr=Inherit: Same as first input
  is : Outport  InitialOutput=0
  wires:
  Mux3/1 -> is/1
  Fcn1/1 -> Mux3/2, Sum/1
  Fcn/1 -> Mux3/1, Sum/2
  Sum/1 -> Mux3/3
  iq,id/1 -> Mux1/2
  s,c/1 -> Mux1/1
  Mux1/1 -> Fcn1/1, Fcn/1

== system electrical_model/Subsystem1/Electrical model2/Gate Pulse Translation for min sw/v0 ==
  In1 : Inport
  Action Port : ActionPort  ActionType=else
  Out1 : Outport
  wires:
  In1/1 -> Out1/1

== system electrical_model/Subsystem1/Electrical model2/Gate Pulse Translation for min sw/v1 ==
  In1 : Inport
  Action Port : ActionPort  ActionType=then
  Out1 : Outport
  wires:
  In1/1 -> Out1/1

== system electrical_model/Subsystem1/Electrical model2/Gate Pulse Translation for min sw/v2 ==
  In1 : Inport
  Action Port : ActionPort  ActionType=elseif
  Out1 : Outport
  wires:
  In1/1 -> Out1/1

== system electrical_model/Subsystem1/Electrical model2/Gate Pulse Translation for min sw/v3 ==
  In1 : Inport
  Action Port : ActionPort  ActionType=elseif
  Out1 : Outport
  wires:
  In1/1 -> Out1/1

== system electrical_model/Subsystem1/Electrical model2/Gate Pulse Translation for min sw/v4 ==
  In1 : Inport
  Action Port : ActionPort  ActionType=elseif
  Out1 : Outport
  wires:
  In1/1 -> Out1/1

== system electrical_model/Subsystem1/Electrical model2/Gate Pulse Translation for min sw/v5 ==
  In1 : Inport
  Action Port : ActionPort  ActionType=elseif
  Out1 : Outport
  wires:
  In1/1 -> Out1/1

== system electrical_model/Subsystem1/Electrical model2/Gate Pulse Translation for min sw/v6 ==
  In1 : Inport
  Action Port : ActionPort  ActionType=elseif
  Out1 : Outport
  wires:
  In1/1 -> Out1/1

== system electrical_model/Subsystem1/Electrical model2/Gate Pulse Translation for min sw/v7 ==
  In1 : Inport
  Action Port : ActionPort  ActionType=elseif
  Out1 : Outport
  wires:
  In1/1 -> Out1/1

== system electrical_model/Subsystem1/Electrical model2/Hall effect sensor/Angle converter ==
  note: This subsystem convert 0,infinite angle to -180,180 angle
  the : Inport
  Trigonometric Function : Trigonometry
  Trigonometric Function1 : Trigonometry  Operator=cos
  Trigonometric Function2 : Trigonometry  Operator=atan2
  rad2deg : Gain  Gain=180/pi  SaturateOnIntegerOverflow=on  OutDataTypeStr=Inherit: Same as input  ParamDataTypeStr=Inherit: Same as input
  the_deg : Outport
  wires:
  the/1 -> Trigonometric Function/1, Trigonometric Function1/1
  Trigonometric Function/1 -> Trigonometric Function2/1
  Trigonometric Function1/1 -> Trigonometric Function2/2
  Trigonometric Function2/1 -> rad2deg/1
  rad2deg/1 -> the_deg/1

== system electrical_model/Subsystem1/Electrical model2/Select Min Cost/v7 and v1 ==
  In1 : Inport
  Action Port : ActionPort  ActionType=elseif
  Out1 : Outport
  wires:
  In1/1 -> Out1/1

== system electrical_model/Subsystem1/Electrical model2/Select Min Cost/v7 and v2 ==
  In1 : Inport
  Action Port : ActionPort  ActionType=then
  Out1 : Outport
  wires:
  In1/1 -> Out1/1

== system electrical_model/Subsystem1/Electrical model2/Voltage Vector Table/v1 ==
  In1 : Inport
  Action Port : ActionPort  ActionType=then
  Out1 : Outport
  wires:
  In1/1 -> Out1/1

== system electrical_model/Subsystem1/Electrical model2/Voltage Vector Table/v2 ==
  In1 : Inport
  Action Port : ActionPort  ActionType=elseif
  Out1 : Outport
  wires:
  In1/1 -> Out1/1

== system electrical_model/Subsystem1/Electrical model2/Voltage Vector Table/v3 ==
  In1 : Inport
  Action Port : ActionPort  ActionType=elseif
  Out1 : Outport
  wires:
  In1/1 -> Out1/1

== system electrical_model/Subsystem1/Electrical model2/Voltage Vector Table/v4 ==
  In1 : Inport
  Action Port : ActionPort  ActionType=elseif
  Out1 : Outport
  wires:
  In1/1 -> Out1/1

== system electrical_model/Subsystem1/Electrical model2/Voltage Vector Table/v5 ==
  In1 : Inport
  Action Port : ActionPort  ActionType=elseif
  Out1 : Outport
  wires:
  In1/1 -> Out1/1

== system electrical_model/Subsystem1/Electrical model2/Voltage Vector Table/v6 ==
  In1 : Inport
  Action Port : ActionPort  ActionType=elseif
  Out1 : Outport
  wires:
  In1/1 -> Out1/1

== system electrical_model/Subsystem1/Electrical model2/Voltage Vector Table/v7 and v0 ==
  In1 : Inport
  Action Port : ActionPort  ActionType=elseif
  Out1 : Outport
  wires:
  In1/1 -> Out1/1

== system electrical_model/Subsystem1/Electrical model2/iq,id1/id ==
  iq : Inport
  we : Inport  Port=2
  vd : Inport  Port=3
  1/Ld : Gain  Gain=1/Li  SaturateOnIntegerOverflow=on  OutDataTypeStr=Inherit: Same as input  ParamDataTypeStr=Inherit: Same as input
  Discrete-Time Integrator : DiscreteIntegrator  SampleTime=Ts  ICPrevOutput=DiscIntNeverNeededParam  ICPrevScaledInput=DiscIntNeverNeededParam
  Product : Product  SaturateOnIntegerOverflow=on  InputSameDT=on  OutDataTypeStr=Inherit: Same as first input
  R/Ld : Gain  Gain=ri/Li  SaturateOnIntegerOverflow=on  OutDataTypeStr=Inherit: Same as input  ParamDataTypeStr=Inherit: Same as input
  Sum : Sum  Inputs=-++  SaturateOnIntegerOverflow=on  InputSameDT=on  OutDataTypeStr=Inherit: Same as first input
  id : Outport  InitialOutput=0
  wires:
  iq/1 -> Product/2
  we/1 -> Product/1
  vd/1 -> 1/Ld/1
  Discrete-Time Integrator/1 -> id/1, R/Ld/1
  Sum/1 -> Discrete-Time Integrator/1
  Product/1 -> Sum/3
  R/Ld/1 -> Sum/1
  1/Ld/1 -> Sum/2

== system electrical_model/Subsystem1/Electrical model2/iq,id1/iq ==
  vq : Inport
  we : Inport  Port=2
  id : Inport  Port=3
  1/Lq : Gain  Gain=1/Li  SaturateOnIntegerOverflow=on  OutDataTypeStr=Inherit: Same as input  ParamDataTypeStr=Inherit: Same as input
  Discrete-Time Integrator : DiscreteIntegrator  SampleTime=Ts  ICPrevOutput=DiscIntNeverNeededParam  ICPrevScaledInput=DiscIntNeverNeededParam
  Product1 : Product  SaturateOnIntegerOverflow=on  InputSameDT=on  OutDataTypeStr=Inherit: Same as first input
  R/Lq : Gain  Gain=ri/Li  SaturateOnIntegerOverflow=on  OutDataTypeStr=Inherit: Same as input  ParamDataTypeStr=Inherit: Same as input
  Sum1 : Sum  Inputs=---+  SaturateOnIntegerOverflow=on  InputSameDT=on  OutDataTypeStr=Inherit: Same as first input
  lam/Lq : Gain  Gain=F/Li  SaturateOnIntegerOverflow=on  OutDataTypeStr=Inherit: Same as input  ParamDataTypeStr=Inherit: Same as input
  iq : Outport  InitialOutput=0
  wires:
  Discrete-Time Integrator/1 -> iq/1, R/Lq/1
  we/1 -> lam/Lq/1, Product1/2
  vq/1 -> 1/Lq/1
  id/1 -> Product1/1
  1/Lq/1 -> Sum1/4
  Sum1/1 -> Discrete-Time Integrator/1
  lam/Lq/1 -> Sum1/3
  Product1/1 -> Sum1/2
  R/Lq/1 -> Sum1/1

== system electrical_model/Subsystem/Other/Electrical model/Hall effect sensor/Angle converter ==
  note: This subsystem convert 0,infinite angle to -180,180 angle
  the : Inport
  Trigonometric Function : Trigonometry
  Trigonometric Function1 : Trigonometry  Operator=cos
  Trigonometric Function2 : Trigonometry  Operator=atan2
  rad2deg : Gain  Gain=180/pi  SaturateOnIntegerOverflow=on  OutDataTypeStr=Inherit: Same as input  ParamDataTypeStr=Inherit: Same as input
  the_deg : Outport
  wires:
  the/1 -> Trigonometric Function/1, Trigonometric Function1/1
  Trigonometric Function/1 -> Trigonometric Function2/1
  Trigonometric Function1/1 -> Trigonometric Function2/2
  Trigonometric Function2/1 -> rad2deg/1
  rad2deg/1 -> the_deg/1

== system electrical_model/Subsystem/Other/Electrical model/iq,id/id ==
  vd : Inport
  we : Inport  Port=2
  iq : Inport  Port=3
  1-Ri/Li*Ts : Gain  Gain=1-ri/Li*Ts  SaturateOnIntegerOverflow=on  OutDataTypeStr=Inherit: Same as input  ParamDataTypeStr=Inherit: Same as input
  Product1 : Product  SaturateOnIntegerOverflow=on  InputSameDT=on  OutDataTypeStr=Inherit: Same as first input
  Sum1 : Sum  Inputs=-++  SaturateOnIntegerOverflow=on  InputSameDT=on  OutDataTypeStr=Inherit: Same as first input
  Ts : Gain  Gain=Ts  SaturateOnIntegerOverflow=on  OutDataTypeStr=Inherit: Same as input  ParamDataTypeStr=Inherit: Same as input
  Ts/Li : Gain  Gain=Ts/Li  SaturateOnIntegerOverflow=on  OutDataTypeStr=Inherit: Same as input  ParamDataTypeStr=Inherit: Same as input
  Unit Delay : UnitDelay  SampleTime=-1
  id : Outport  InitialOutput=0
  wires:
  1-Ri/Li*Ts/1 -> Sum1/1
  Ts/1 -> Sum1/2
  Sum1/1 -> Unit Delay/1  "idot"
  Product1/1 -> Ts/1
  Ts/Li/1 -> Sum1/3
  iq/1 -> Product1/1
  vd/1 -> Ts/Li/1
  we/1 -> Product1/2
  Unit Delay/1 -> id/1, 1-Ri/Li*Ts/1

== system electrical_model/Subsystem/Other/Electrical model/iq,id/iq ==
  vq : Inport
  we : Inport  Port=2
  id : Inport  Port=3
  1-Ri/Li*Ts : Gain  Gain=1-ri/Li*Ts  SaturateOnIntegerOverflow=on  OutDataTypeStr=Inherit: Same as input  ParamDataTypeStr=Inherit: Same as input
  Product1 : Product  SaturateOnIntegerOverflow=on  InputSameDT=on  OutDataTypeStr=Inherit: Same as first input
  Sum1 : Sum  Inputs=--+  SaturateOnIntegerOverflow=on  InputSameDT=on  OutDataTypeStr=Inherit: Same as first input
  Ts : Gain  Gain=Ts  SaturateOnIntegerOverflow=on  OutDataTypeStr=Inherit: Same as input  ParamDataTypeStr=Inherit: Same as input
  Ts/Li : Gain  Gain=Ts/Li  SaturateOnIntegerOverflow=on  OutDataTypeStr=Inherit: Same as input  ParamDataTypeStr=Inherit: Same as input
  Unit Delay : UnitDelay  SampleTime=-1
  iq : Outport  InitialOutput=0
  wires:
  1-Ri/Li*Ts/1 -> Sum1/1
  Ts/1 -> Sum1/2
  Sum1/1 -> Unit Delay/1  "idot"
  Product1/1 -> Ts/1
  Ts/Li/1 -> Sum1/3
  id/1 -> Product1/1
  vq/1 -> Ts/Li/1
  we/1 -> Product1/2
  Unit Delay/1 -> 1-Ri/Li*Ts/1, iq/1

== matlab function electrical_model/Subsystem1/Electrical model2/current and power prediction/cost function ==
  data: u input; P output; Iqd_next output; cost output
function [P,Iqd_next,cost] = fcn(u)
%%initialization

N=22.5; %rpm rated speed,the generator will works at its maximum rated speed
r=22.9;  %m radius of the rotor
Cp_op=0.43;
Cp_min=0.32;
Cp_max=0.52; %min and max values of the power coefficient change the reference power of the generator if to beused


F=1;
ri=0.1;  % Grid side converter harmonic filter resistance
Ts=1e-4;%data sampling time
step_size=1/Ts;

w_g=N*pi/30; % mechanical speed
T=1/(2*pi*w_g);
% generator is 26 pole pair machine hence: w_g_e=w_g*26; the electrical
% speed equivalent
Theta=zeros();
for k=0:1:(step_size-1)
    Theta(k+1)=k*Ts*w_g;
end

Li= 0.16e-3; % Grid side converter harmonic filter inductance
k=1;
xVec=zeros();
yVec=zeros();
Usol=zeros();

%%

A11=(1-ri*Ts)/Li;
A12=w_g*Ts;
A21=-A12;
A22=A11;

B11=Ts/Li;
B22=B11;
B12=0;
B21=0;

v_dg=100;
v_qg=100;

%% Voltage vectoral representation in dq frame

A=[A11 A12; A21 A22];
B=[B11 B12; B21 B22];
C=[v_dg v_qg];
D=0;



%% Optimal control solution for $N = 4$

G = [zeros(2,2) zeros(2,2) zeros(2,2) zeros(2,2); B zeros(2,2) zeros(2,2) zeros(2,2); ...
    A*B B zeros(2,2) zeros(2,2); A^2*B A*B B zeros(2,2); A^3*B A^2*B A*B B];
H = [eye(2); A; A^2; A^3; A^4];
%Q = C'*C;
R = .01;
Q = eye(2);

Pinf = dare(A,B,Q,R,zeros(2,2),eye(2) );
Kinf = inv(R+B'*Pinf*B)*B'*Pinf*A;

P = dlyap( (A-B*Kinf)',Q+Kinf'*R*Kinf);
Qf = P;
Qbar = blkdiag(Q,Q,Q,Q,Qf);
Rbar = blkdiag(R,R,R,R);
M = G'*Qbar*G + Rbar;

%% min-max

umin = -Inf;
umax = Inf;
umin = -4;
umax = 4;
lb = [umin;umin;umin;umin];
ub = [umax;umax;umax;umax];

%%

xVec(1) = x0;
yVec(1) = C*x0;
uVec = [];
xVec(k)=u;

    alpha = G'*Qbar*H*xVec(:,k);
    Usol = quadprog(M,alpha',[],[],[],[],lb,ub);
    uVec(k) = Usol(1);
    xVec(k+1) = A*xVec(k) + B*uVec(k);
    yVec(k+1) = C*xVec(k+1);

    k=k+1;


P=yVec(k+1);
Iqd_next=xVec(k+1) ;
end
